simulink model "test_file"  (R2019b)
settings: Solver=VariableStepAuto  StartTime=0.0  StopTime=10.0  RelTol=1e-3
settings Model: Creator=dt1005418  LastModifiedBy=dt1005418

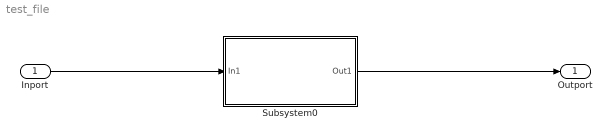
== system test_file ==
  Inport : Inport
  Subsystem0 : Subsystem  mask{gainVal0=1, gainVal1=0}
      mask prompts: gainVal0 "gain value:"; gainVal1 "more gains:"
  Outport : Outport
  wires:
  Inport/1 -> Subsystem0/1(In1)
  Subsystem0/1(Out1) -> Outport/1

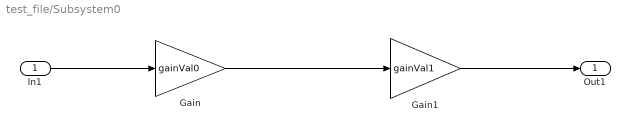
== system test_file/Subsystem0 ==
  In1 : Inport
  Gain : Gain  Gain=gainVal0
  Gain1 : Gain  Gain=gainVal1
  Out1 : Outport
  wires:
  In1/1 -> Gain/1
  Gain/1 -> Gain1/1
  Gain1/1 -> Out1/1
